simulink library "NonlinearModel_Lib"  (Simulink 8.0)
settings: Solver=ode45  StartTime=0.0  StopTime=10.0  RelTol=1e-3
values from neighbouring files (symbols this model uses):
  AC = miniMUTT_rigid_config    [UAV_config.m]    (also in UAV_modelconfig.mat = )
undefined symbols (not defined in the file or in its folder): m, s
undefined symbols (not defined in the file): TrimCondition
libraries: aerolib6dofsys x4, aerolibconvert2 x2, simulink x1, aerolibutil x1, AuxEq_Lib x1, Aero_Lib x1, Propulsion_Lib x1, Gravity_Lib x1
settings Model: Creator=Paul Freeman  LastModifiedBy=singh461

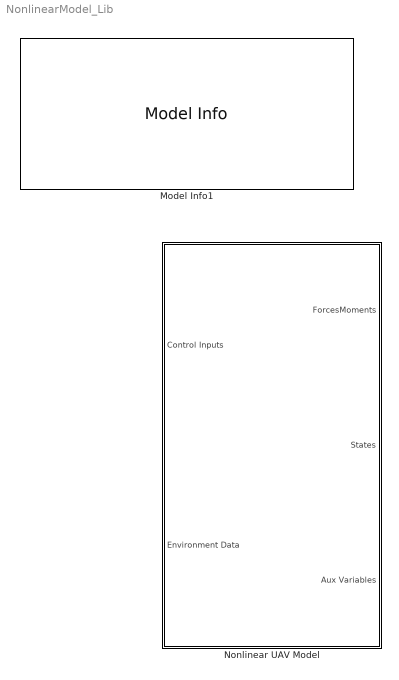
== system NonlinearModel_Lib ==
  Model Info1 : simulink/Model-Wide Utilities/Model Info  InitialBlockCM=None  BlockCM=None  Frame=on  DisplayStringWithTags=|  HorizontalTextAlignment=Left  LeftAlignmentValue=0.02  SourceBlockDiagram=NonlinearModel_Lib  TagMaxNumber=20
      | MODEL INFORMATION
      | UAV Nonlinear Model Library
      | 
      | University of Minnesota
      | Aerospace Engineering and Mechanics
      | Copyright 2011 Regents of the University of Minnesota. All rights reserved.
      | 
      | == SVN Info ==
      | Last modified by %<LastModifiedBy> on %<LastModificationDate>
  Nonlinear UAV Model : Subsystem

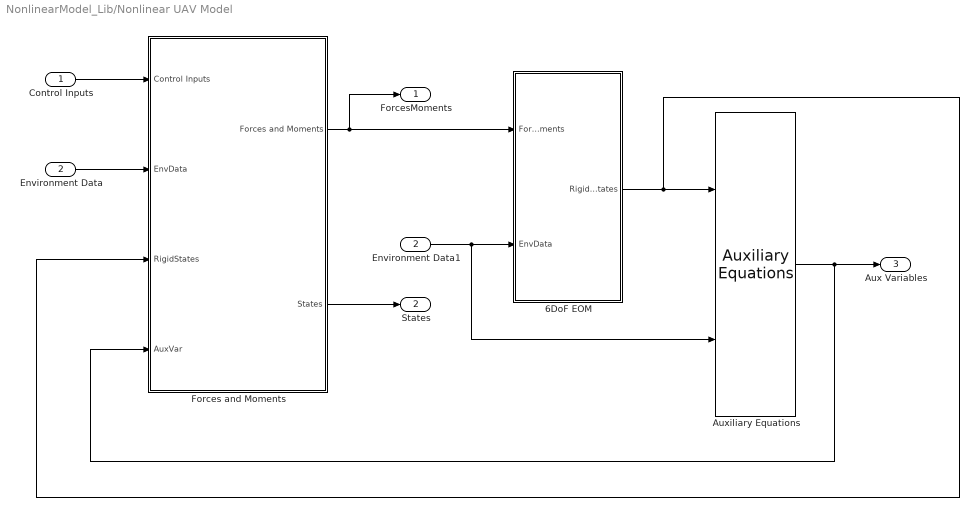
== system NonlinearModel_Lib/Nonlinear UAV Model ==
  Control Inputs : Inport
  Environment Data : Inport  Port=2
  6DoF EOM : Subsystem  mask(6DoF EoM (Body Axis)){units=Metric (MKS), mtype=Fixed, rep=Euler Angles, xme_0=TrimCondition.InertialIni, Vm_0=TrimCondition.VelocitiesIni, eul_0=TrimCondition.AttitudeIni, pm_0=TrimCondition.RatesIni, mass_0=AC.Mass, mass_e=0.5, mass_f=2.0, inertia=AC.Inertia.Matrix, inertia_e=eye(3), inertia_f=2*eye(3), k_quat=1.0}
      mask prompts: mtype "Mass type:"; rep "Representation:"; xme_0 "Initial position in inertial axes [Xe,Ye,Ze]:"; Vm_0 "Initial velocity in body axes [U,v,w]:"; eul_0 "Initial Euler orientation [roll, pitch, yaw]:"; pm_0 "Initial body rotation rates [p,q,r]:"; mass_0 "Initial mass:"; mass_e "Empty mass:"; mass_f "Full mass:"; inertia_e "Empty inertia matrix:"; inertia_f "Full inertia matrix:"; k_quat "Gain for quaternion normalization:"
      mask help:
      | Integrate the six-degrees-of-freedom equations of motion in body axis.
      |
      | This block has been modified from the original Aerospace Blockset
      | implementation. The inertial position vector (Xe) is no longer computed.
      | The original block did not have a way to add steady state winds to the
      | inertial velocities (Ve) prior to integrating to get Xe. Therefore, this
      | step is performed in the Auxiliary Equations block.
      mask Help: eval('asbhelp(''sixdof_euler_angles'')');
      mask TypeOptions units: Metric (MKS) | English (Velocity in ft/s) | English (Velocity in kts)
      mask TypeOptions mtype: Fixed | Simple Variable | Custom Variable
      mask Callback mtype: aeroicon('aeroblk6dofbody');
      mask TypeOptions rep: Euler Angles | Quaternion
      mask Callback rep: aeroicon('aeroblk6dofbody');
  Auxiliary Equations : AuxEq_Lib/Auxiliary Equations
  Environment Data1 : InportShadow  Port=2
  Forces and Moments : Subsystem
  ForcesMoments : Outport
  States : Outport  Port=2
  Aux Variables : Outport  Port=3
  wires:
  Forces and Moments/1(Forces and Moments) -> ForcesMoments/1, 6DoF EOM/1(Forces and Moments)
  Control Inputs/1 -> Forces and Moments/1(Control Inputs)
  6DoF EOM/1(RigidStates) -> Auxiliary Equations/1, Forces and Moments/3(RigidStates)
  Auxiliary Equations/1 -> Forces and Moments/4(AuxVar), Aux Variables/1
  Environment Data/1 -> Forces and Moments/2(EnvData)
  Environment Data1/1 -> Auxiliary Equations/2, 6DoF EOM/2(EnvData)
  Forces and Moments/2(States) -> States/1

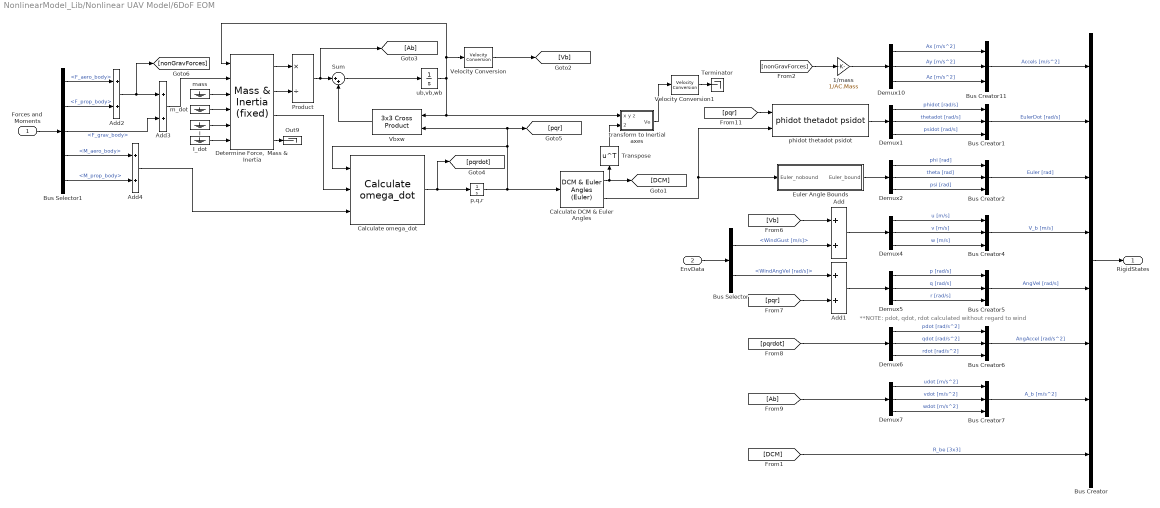
== system NonlinearModel_Lib/Nonlinear UAV Model/6DoF EOM ==
  note: **NOTE: pdot, qdot, rdot calculated without regard to wind
  Forces and Moments : Inport
  EnvData : Inport  Port=2
  1/mass : Gain  Gain=1/AC.Mass
  Add{,1..4} (5 alike) : Sum
  Bus Creator{1..2,4..7,11} (7 alike) : BusCreator  Inputs=3
  Bus Selector : BusSelector  OutputSignals=WindGust [m/s],WindAngVel [rad/s]
  Bus Selector1 : BusSelector  OutputSignals=AeroLoads.F_aero_body,F_prop_body,F_grav_body,AeroLoads.M_aero_body,M_prop_body
  Bus Creator : BusCreator  Inputs=8
  Calculate DCM & Euler Angles : aerolib6dofsys/DCM & Euler Angles (Euler)  SystemSampleTime=-1
  Calculate omega_dot : aerolib6dofsys/Calculate omega_dot
  Demux{1..2,4..7,10} (7 alike) : Demux  Outputs=3
  "Determine Force,  Mass & Inertia" : aerolib6dofsys/Mass & Inertia (fixed)  SystemSampleTime=-1
  Euler Angle Bounds : Subsystem
  I : Ground
  I_dot : Ground
  Out9 : Terminator
  Product : Product  Inputs=*/  SaturateOnIntegerOverflow=on  OutDataTypeStr=Inherit: Same as first input
  Sum : Sum  Inputs=|++  SaturateOnIntegerOverflow=on
  Terminator : Terminator
  Transpose : Math  Operator=transpose  SaturateOnIntegerOverflow=on
  Vbxw : aerolibutil/3x3 Cross Product
  Velocity Conversion : aerolibconvert2/Velocity Conversion  IU=m/s  OU=m/s
  Velocity Conversion1 : aerolibconvert2/Velocity Conversion  IU=m/s  OU=m/s
  m_dot : Ground
  mass : Ground
  "p,q,r " : Integrator  InitialCondition=pm_0
  phidot thetadot psidot : aerolib6dofsys/DCM & Euler Angles (Euler)/phidot thetadot psidot
  "transform to Inertial axes " : Subsystem  mask(Vector Transformation){}
      mask Display: disp('L_EB')
  ub,vb,wb : Integrator  InitialCondition=convvel(Vm_0,'m/s','m/s')
  RigidStates : Outport
  wires:
  "Determine Force,  Mass & Inertia"/1 -> Product/1
  I_dot/1 -> "Determine Force,  Mass & Inertia"/6
  I/1 -> "Determine Force,  Mass & Inertia"/5
  Calculate omega_dot/1 -> [pqrdot], "p,q,r "/1
  "Determine Force,  Mass & Inertia"/4 -> Out9/1
  m_dot/1 -> "Determine Force,  Mass & Inertia"/4
  "Determine Force,  Mass & Inertia"/2 -> Product/2
  mass/1 -> "Determine Force,  Mass & Inertia"/3
  Transpose/1 -> "transform to Inertial axes "/2(transform coefficients)
  Calculate DCM & Euler Angles/1 -> [DCM], Transpose/1
  Product/1 -> [Ab], Sum/1
  "p,q,r "/1 -> Calculate omega_dot/1, [pqr], Vbxw/2, Calculate DCM & Euler Angles/1
  "transform to Inertial axes "/1(Ve) -> Velocity Conversion1/1
  Sum/1 -> ub,vb,wb/1
  ub,vb,wb/1 -> "Determine Force,  Mass & Inertia"/1, Velocity Conversion/1, Vbxw/1, "transform to Inertial axes "/1(x y z)
  Vbxw/1 -> Sum/2
  "Determine Force,  Mass & Inertia"/3 -> Calculate omega_dot/2
  Velocity Conversion/1 -> [Vb]
  Velocity Conversion1/1 -> Terminator/1
  Bus Creator/1 -> RigidStates/1
  EnvData/1 -> Bus Selector/1
  Bus Selector/1 -> Add/2  "<WindGust [m/s]>"
  Bus Selector/2 -> Add1/1  "<WindAngVel [rad/s]>"
  [Vb] -> Add/1
  Add/1 -> Demux4/1
  Demux4/3 -> Bus Creator4/3  "w [m/s]"
  Demux4/2 -> Bus Creator4/2  "v [m/s]"
  Demux4/1 -> Bus Creator4/1  "u [m/s]"
  Bus Creator4/1 -> Bus Creator/4  "V_b [m/s]"
  [pqr] -> Add1/2
  Demux5/3 -> Bus Creator5/3  "r [rad/s]"
  Demux5/2 -> Bus Creator5/2  "q [rad/s]"
  Demux5/1 -> Bus Creator5/1  "p [rad/s]"
  Bus Creator5/1 -> Bus Creator/5  "AngVel [rad/s]"
  Add1/1 -> Demux5/1
  [pqrdot] -> Demux6/1
  Demux6/3 -> Bus Creator6/3  "rdot [rad/s^2]"
  Demux6/2 -> Bus Creator6/2  "qdot [rad/s^2]"
  Demux6/1 -> Bus Creator6/1  "pdot [rad/s^2]"
  Bus Creator6/1 -> Bus Creator/6  "AngAccel [rad/s^2]"
  [Ab] -> Demux7/1
  Demux7/3 -> Bus Creator7/3  "wdot [m/s^2]"
  Demux7/2 -> Bus Creator7/2  "vdot [m/s^2]"
  Demux7/1 -> Bus Creator7/1  "udot [m/s^2]"
  Bus Creator7/1 -> Bus Creator/7  "A_b [m/s^2]"
  Demux1/3 -> Bus Creator1/3  "psidot [rad/s]"
  Demux1/2 -> Bus Creator1/2  "thetadot [rad/s]"
  Demux1/1 -> Bus Creator1/1  "phidot [rad/s]"
  Bus Creator1/1 -> Bus Creator/2  "EulerDot [rad/s]"
  phidot thetadot psidot/1 -> Demux1/1
  [pqr] -> phidot thetadot psidot/1
  Calculate DCM & Euler Angles/2 -> Euler Angle Bounds/1(Euler_nobound), phidot thetadot psidot/2
  Demux2/3 -> Bus Creator2/3  "psi [rad]"
  Demux2/2 -> Bus Creator2/2  "theta [rad]"
  Demux2/1 -> Bus Creator2/1  "phi [rad]"
  Bus Creator2/1 -> Bus Creator/3  "Euler [rad]"
  Euler Angle Bounds/1(Euler_bound) -> Demux2/1
  Bus Creator11/1 -> Bus Creator/1  "Accels [m/s^2]"
  [nonGravForces] -> 1/mass/1
  1/mass/1 -> Demux10/1
  Demux10/1 -> Bus Creator11/1  "Ax [m/s^2]"
  Demux10/2 -> Bus Creator11/2  "Ay [m/s^2]"
  Demux10/3 -> Bus Creator11/3  "Az [m/s^2]"
  [DCM] -> Bus Creator/8  "R_be [3x3]"
  Forces and Moments/1 -> Bus Selector1/1
  Bus Selector1/1 -> Add2/1  "<F_aero_body>"
  Bus Selector1/2 -> Add2/2  "<F_prop_body>"
  Add2/1 -> [nonGravForces], Add3/1
  Bus Selector1/3 -> Add3/2  "<F_grav_body>"
  Add3/1 -> "Determine Force,  Mass & Inertia"/2
  Bus Selector1/4 -> Add4/1  "<M_aero_body>"
  Bus Selector1/5 -> Add4/2  "<M_prop_body>"
  Add4/1 -> Calculate omega_dot/3

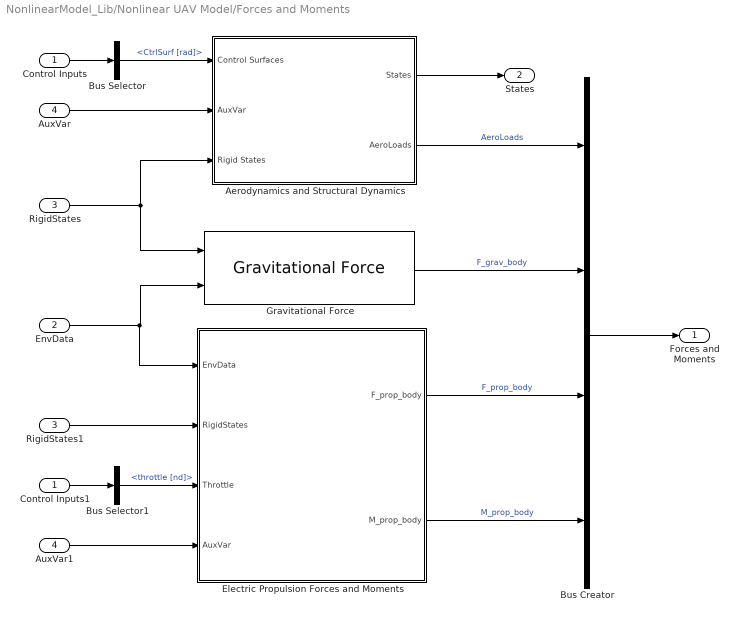
== system NonlinearModel_Lib/Nonlinear UAV Model/Forces and Moments ==
  Control Inputs : Inport
  EnvData : Inport  Port=2
  RigidStates : Inport  Port=3
  AuxVar : Inport  Port=4
  Aerodynamics and Structural Dynamics : Subsystem  BlockChoice=rigid AC  mask{aircraft=AC.aircraft}
      mask prompts: aircraft "Aircraft model:"
      mask help: Select aerodynamic model based on AC.aircraft variable
      mask init:
      | pathname = gcb;
      | 
      | switch lower(aircraft)
      |     case 'ultrastick120'
      |         set_param(pathname,'BlockChoice','rigid AC');
      |         set_param([pathname '/rigid AC/Aerodynamic Coefficients'],'BlockChoice','UltraStick120');
      | %         set_param([pathname '/UltraStick/Forces and Moments Calculation'],'inputAxes','Stability');
      | %         set_param([pathname '/UltraStick/Forces and Moments Calculation'],'outputMomentAxes','Stability');
      |     case 'ultrastick25e'
      |         set_param(pathname,'BlockChoice','rigid AC');
      |         set_param([pathname '/rigid AC/Aerodynamic Coefficients'],'BlockChoice','UltraStick25e');
      | %         set_param([pathname '/UltraStick/Forces and Moments Calculation'],'inputAxes','Wind');
      | %         set_param([pathname '/UltraStick/Forces and Moments Calculation'],'outputMomentAxes','Wind');
      |     case 'rigid_minimutt'
      |         set_param(pathname,'BlockChoice','rigid AC');
      |         set_param([pathname '/rigid AC/Aerodynamic Coefficients'],'BlockChoice','rigid miniMUTT');
      | %         set_param(pathname,'BlockChoice','old');
      |     
      |     case 'minimutt'
      |          set_param(pathname,'BlockChoice','miniMUTT');
      |         
      | end
      settings: AttributesFormatString=%<BlockChoice>  TemplateBlock=Aero_Lib/Aerodynamics and Structural Dynamics  MemberBlocks=miniMUTT,old,rigid AC
  AuxVar1 : InportShadow  Port=4
  Bus Selector1 : BusSelector  OutputSignals=throttle [nd]
  Bus Creator : BusCreator
  Bus Selector : BusSelector  OutputSignals=CtrlSurf [rad]
  Control Inputs1 : InportShadow
  Electric Propulsion Forces and Moments : Subsystem  BlockChoice=miniMUTT  mask{aircraft=AC.aircraft}
      mask prompts: aircraft "Aircraft type:"
      mask init:
      | pathname = gcb;
      | 
      | switch lower(aircraft)
      |     case 'ultrastick120'
      |         set_param(pathname,'BlockChoice','UltraStick');
      |     case 'ultrastick25e'
      |         set_param(pathname,'BlockChoice','UltraStick');
      |     case 'minimutt'
      |         set_param(pathname,'BlockChoice','miniMUTT');
      | end
      settings: AttributesFormatString=%<BlockChoice>  TemplateBlock=Propulsion_Lib/Electric Propulsion Forces and Moments  MemberBlocks=UltraStick,miniMUTT
  "Gravitational Force " : Gravity_Lib/Gravitational Force 
  RigidStates1 : InportShadow  Port=3
  Forces and Moments : Outport
  States : Outport  Port=2
  wires:
  Bus Selector/1 -> Aerodynamics and Structural Dynamics/1(Control Surfaces)  "<CtrlSurf [rad]>"
  Control Inputs1/1 -> Bus Selector1/1
  EnvData/1 -> Electric Propulsion Forces and Moments/1(EnvData), "Gravitational Force "/2
  Bus Selector1/1 -> Electric Propulsion Forces and Moments/3(Throttle)  "<throttle [nd]>"
  Aerodynamics and Structural Dynamics/1(States) -> States/1
  Aerodynamics and Structural Dynamics/2(AeroLoads) -> Bus Creator/1  "AeroLoads"
  "Gravitational Force "/1 -> Bus Creator/2  "F_grav_body"
  Bus Creator/1 -> Forces and Moments/1
  AuxVar/1 -> Aerodynamics and Structural Dynamics/2(AuxVar)
  RigidStates/1 -> Aerodynamics and Structural Dynamics/3(Rigid States), "Gravitational Force "/1
  Control Inputs/1 -> Bus Selector/1
  RigidStates1/1 -> Electric Propulsion Forces and Moments/2(RigidStates)
  AuxVar1/1 -> Electric Propulsion Forces and Moments/4(AuxVar)
  Electric Propulsion Forces and Moments/2(M_prop_body) -> Bus Creator/4  "M_prop_body"
  Electric Propulsion Forces and Moments/1(F_prop_body) -> Bus Creator/3  "F_prop_body"

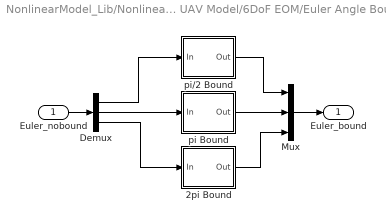
== system NonlinearModel_Lib/Nonlinear UAV Model/6DoF EOM/Euler Angle Bounds ==
  Euler_nobound : Inport
  2pi Bound : Subsystem
  Demux : Demux  Outputs=3
  Mux : Mux  Inputs=3
  pi Bound : Subsystem
  pi/2 Bound : Subsystem
  Euler_bound : Outport
  wires:
  pi Bound/1(Out) -> Mux/2
  pi/2 Bound/1(Out) -> Mux/1
  Mux/1 -> Euler_bound/1
  Euler_nobound/1 -> Demux/1
  Demux/1 -> pi/2 Bound/1(In)
  Demux/2 -> pi Bound/1(In)
  Demux/3 -> 2pi Bound/1(In)
  2pi Bound/1(Out) -> Mux/3

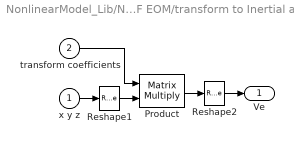
== system NonlinearModel_Lib/Nonlinear UAV Model/6DoF EOM/transform to Inertial axes  ==
  x y z : Inport
  transform coefficients : Inport  Port=2
  Product : Product  Multiplication=Matrix(*)  SaturateOnIntegerOverflow=on  InputSameDT=on  OutDataTypeStr=Inherit: Same as first input
  Reshape1 : Reshape  OutputDimensionality=Column vector (2-D)
  Reshape2 : Reshape
  Ve : Outport
  wires:
  Reshape2/1 -> Ve/1
  Reshape1/1 -> Product/2
  x y z/1 -> Reshape1/1
  transform coefficients/1 -> Product/1
  Product/1 -> Reshape2/1

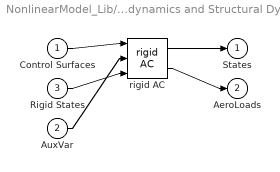
== system NonlinearModel_Lib/Nonlinear UAV Model/Forces and Moments/Aerodynamics and Structural Dynamics ==
  Control Surfaces : Inport
  AuxVar : Inport  Port=2
  Rigid States : Inport  Port=3
  rigid AC : Aero_Lib/rigid AC  aircraft=AC.aircraft
      link override Aerodynamic Coefficients: BlockChoice=rigid miniMUTT
  States : Outport
  AeroLoads : Outport  Port=2
  wires:
  rigid AC/2 -> AeroLoads/1
  rigid AC/1 -> States/1
  Rigid States/1 -> rigid AC/3
  AuxVar/1 -> rigid AC/2
  Control Surfaces/1 -> rigid AC/1

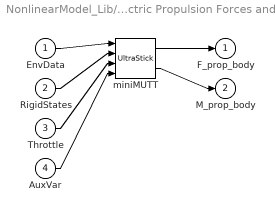
== system NonlinearModel_Lib/Nonlinear UAV Model/Forces and Moments/Electric Propulsion Forces and Moments ==
  EnvData : Inport
  RigidStates : Inport  Port=2
  Throttle : Inport  Port=3
  AuxVar : Inport  Port=4
  miniMUTT : Propulsion_Lib/UltraStick
  F_prop_body : Outport
  M_prop_body : Outport  Port=2
  wires:
  miniMUTT/2 -> M_prop_body/1
  miniMUTT/1 -> F_prop_body/1
  AuxVar/1 -> miniMUTT/4
  Throttle/1 -> miniMUTT/3
  RigidStates/1 -> miniMUTT/2
  EnvData/1 -> miniMUTT/1

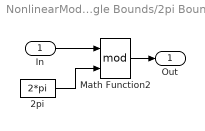
== system NonlinearModel_Lib/Nonlinear UAV Model/6DoF EOM/Euler Angle Bounds/2pi Bound ==
  In : Inport
  2pi : Constant  Value=2*pi
  Math Function2 : Math  Operator=mod  SaturateOnIntegerOverflow=on
  Out : Outport
  wires:
  Math Function2/1 -> Out/1
  2pi/1 -> Math Function2/2
  In/1 -> Math Function2/1

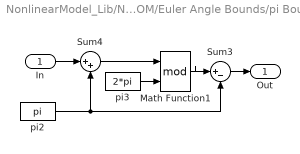
== system NonlinearModel_Lib/Nonlinear UAV Model/6DoF EOM/Euler Angle Bounds/pi Bound ==
  In : Inport
  Math Function1 : Math  Operator=mod  SaturateOnIntegerOverflow=on
  Sum3 : Sum  Inputs=|+-  SaturateOnIntegerOverflow=on  InputSameDT=on  OutDataTypeStr=Inherit: Same as first input
  Sum4 : Sum  Inputs=|++  SaturateOnIntegerOverflow=on  InputSameDT=on  OutDataTypeStr=Inherit: Same as first input
  pi2 : Constant  Value=pi
  pi3 : Constant  Value=2*pi
  Out : Outport
  wires:
  Math Function1/1 -> Sum3/1
  pi3/1 -> Math Function1/2
  In/1 -> Sum4/1
  Sum4/1 -> Math Function1/1
  pi2/1 -> Sum4/2, Sum3/2
  Sum3/1 -> Out/1

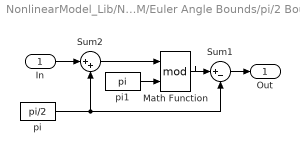
== system NonlinearModel_Lib/Nonlinear UAV Model/6DoF EOM/Euler Angle Bounds/pi/2 Bound ==
  In : Inport
  Math Function : Math  Operator=mod  SaturateOnIntegerOverflow=on
  Sum1 : Sum  Inputs=|+-  SaturateOnIntegerOverflow=on  InputSameDT=on  OutDataTypeStr=Inherit: Same as first input
  Sum2 : Sum  Inputs=|++  SaturateOnIntegerOverflow=on  InputSameDT=on  OutDataTypeStr=Inherit: Same as first input
  pi : Constant  Value=pi/2
  pi1 : Constant  Value=pi
  Out : Outport
  wires:
  Sum1/1 -> Out/1
  pi/1 -> Sum1/2, Sum2/2
  Sum2/1 -> Math Function/1
  In/1 -> Sum2/1
  pi1/1 -> Math Function/2
  Math Function/1 -> Sum1/1
